simulink model "engine_with_clutch"  (R2026a)
settings: Solver=VariableStepAuto  StopTime=10
libraries: fl_lib x13, nesl_utility x12, sdl_lib x1
settings Model: Creator=doyeop  LastModifiedBy=doyeop
settings SolverCC: ZeroCrossAlgorithm=Adaptive
settings DebuggingCC: IgnoredZcDiagnostic=none

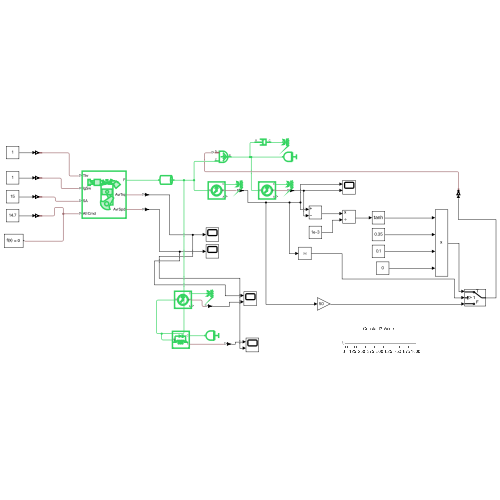
[thumbnail: Simulink's stored preview of the top-level diagram]
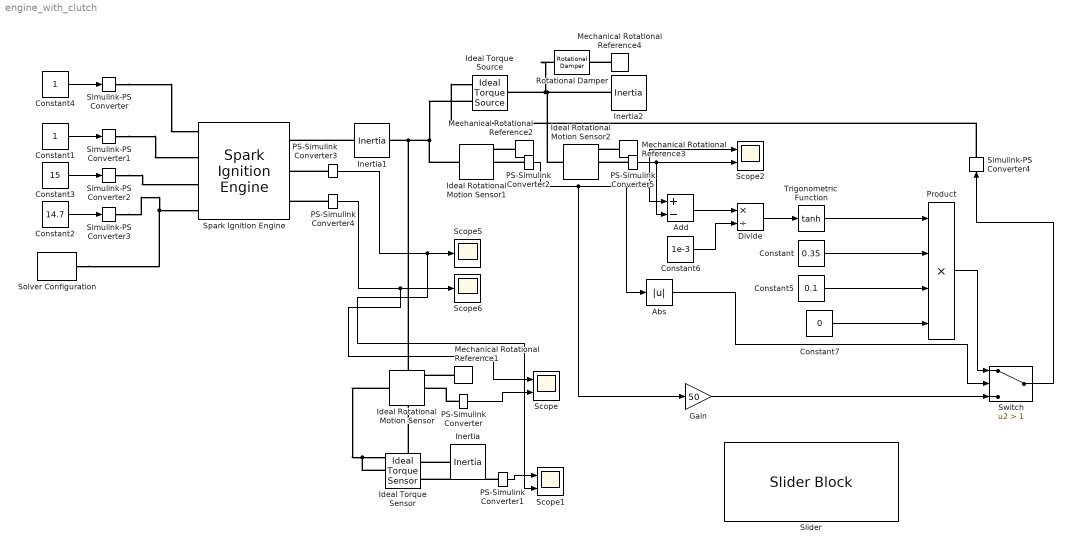
== system engine_with_clutch ==
  Abs : Abs  SaturateOnIntegerOverflow=off
  Add : Sum  Inputs=+-
  Constant : Constant  Value=0.35
  Constant1 : Constant
  Constant2 : Constant  Value=14.7  SampleTime=-1
  Constant3 : Constant  Value=15  SampleTime=-1
  Constant4 : Constant  SampleTime=-1
  Constant5 : Constant  Value=0.1
  Constant6 : Constant  Value=1e-3
  Constant7 : Constant  Value=0
  Divide : Product  Inputs=*/
  Gain : Gain  Gain=50
  Ideal Rotational Motion Sensor : fl_lib/Mechanical/Mechanical Sensors/Ideal Rotational Motion Sensor  reference=foundation.enum.MeasurementReference.difference  acceleration_port=false  velocity_port=true  position_port=true  wrap_angle=false  offset=0 rad
  Ideal Rotational Motion Sensor1 : fl_lib/Mechanical/Mechanical Sensors/Ideal Rotational Motion Sensor  reference=foundation.enum.MeasurementReference.difference  acceleration_port=false  velocity_port=true  position_port=true  wrap_angle=false  offset=0 rad
  Ideal Rotational Motion Sensor2 : fl_lib/Mechanical/Mechanical Sensors/Ideal Rotational Motion Sensor  reference=foundation.enum.MeasurementReference.difference  acceleration_port=false  velocity_port=true  position_port=true  wrap_angle=false  offset=0 rad
  Ideal Torque Sensor : fl_lib/Mechanical/Mechanical Sensors/Ideal Torque Sensor
  Ideal Torque Source : fl_lib/Mechanical/Mechanical Sources/Ideal Torque Source
  Inertia : fl_lib/Mechanical/Rotational Elements/Inertia  inertia=0.1 kg*m^2  num_ports=foundation.enum.numPorts2.one  w_specify=on  w_priority=None  w=0 rpm  w_nominal_specify=off  w_nominal_value=1  w_nominal_unit=rad/s  t_specify=off  t_priority=None  t=0 N*m  t_nominal_specify=off  t_nominal_value=1  t_nominal_unit=N*m
  Inertia1 : fl_lib/Mechanical/Rotational Elements/Inertia  inertia=0.01 kg*m^2  num_ports=foundation.enum.numPorts2.two  w_specify=on  w_priority=High  w=800 rpm  w_nominal_specify=off  w_nominal_value=1  w_nominal_unit=rad/s  t_specify=off  t_priority=None  t=0 N*m  t_nominal_specify=off  t_nominal_value=1  t_nominal_unit=N*m
  Inertia2 : fl_lib/Mechanical/Rotational Elements/Inertia  inertia=0.05 kg*m^2  num_ports=foundation.enum.numPorts2.one  w_specify=on  w_priority=None  w=0 rpm  w_nominal_specify=off  w_nominal_value=1  w_nominal_unit=rad/s  t_specify=off  t_priority=None  t=0 N*m  t_nominal_specify=off  t_nominal_value=1  t_nominal_unit=N*m
  Mechanical Rotational Reference{1..4} (4 alike) : fl_lib/Mechanical/Rotational Elements/Mechanical Rotational Reference
  PS-Simulink Converter{,2,4..5} (4 alike) : nesl_utility/PS-Simulink Converter  PhysicalDomain=network_engine_domain  SubClassName=ps_output  LeftPortType=input  RightPortType=output  PseudoPeriodic=off  Frequencies=[]  VectorFormat=inherit  Unit=rpm  AffineConversion=off
  PS-Simulink Converter1 : nesl_utility/PS-Simulink Converter  PhysicalDomain=network_engine_domain  SubClassName=ps_output  LeftPortType=input  RightPortType=output  PseudoPeriodic=off  Frequencies=[]  VectorFormat=inherit  Unit=N*m  AffineConversion=off
  PS-Simulink Converter3 : nesl_utility/PS-Simulink Converter  PhysicalDomain=network_engine_domain  SubClassName=ps_output  LeftPortType=input  RightPortType=output  PseudoPeriodic=off  Frequencies=[]  VectorFormat=inherit  Unit=N*m  AffineConversion=off
  Product : Product  Inputs=4
  Rotational Damper : fl_lib/Mechanical/Rotational Elements/Rotational Damper  D=0.1 N*m*s/rad  w_specify=off  w_priority=None  w=0 rad/s  w_nominal_specify=off  w_nominal_value=1  w_nominal_unit=rad/s  t_specify=off  t_priority=None  t=0 N*m  t_nominal_specify=off  t_nominal_value=1  t_nominal_unit=N*m
  Scope : Scope  NumInputPorts=2
      settings: ActiveDisplayYMinimum=-2000.3458595498478  ActiveDisplayYMaximum=18003.112735948635
  Scope1 : Scope  NumInputPorts=2
      settings: ActiveDisplayYMinimum=-41.551396950603035  ActiveDisplayYMaximum=102.79160135138113
  Scope2 : Scope  NumInputPorts=2
      settings: ActiveDisplayYMinimum=-1664.2475997401448  ActiveDisplayYMaximum=14978.228397661307  DataLoggingVariableName=ScopeData2
  Scope5 : Scope
      settings: ActiveDisplayYMinimum=-2.7962714720759139  ActiveDisplayYMaximum=25.16644324868323  DataLoggingVariableName=ScopeData5
  Scope6 : Scope
      settings: ActiveDisplayYMinimum=-1506.4519625720234  ActiveDisplayYMaximum=13558.067663148213  DataLoggingVariableName=ScopeData6
  Simulink-PS Converter : nesl_utility/Simulink-PS Converter  PhysicalDomain=network_engine_domain  SubClassName=ps_input  LeftPortType=input  RightPortType=output  PseudoPeriodic=off  Frequencies=[]  NoiseDistribution=none  NoiseParameters=[]  Unit=1  AffineConversion=off  FilteringAndDerivatives=provide  SimscapeFilterOrder=1  InputFilterTimeConstant=0.001  UdotUserProvided=0
  Simulink-PS Converter1 : nesl_utility/Simulink-PS Converter  PhysicalDomain=network_engine_domain  SubClassName=ps_input  LeftPortType=input  RightPortType=output  PseudoPeriodic=off  Frequencies=[]  NoiseDistribution=none  NoiseParameters=[]  Unit=1  AffineConversion=off  FilteringAndDerivatives=provide  SimscapeFilterOrder=1  InputFilterTimeConstant=0.001  UdotUserProvided=0
  Simulink-PS Converter2 : nesl_utility/Simulink-PS Converter  PhysicalDomain=network_engine_domain  SubClassName=ps_input  LeftPortType=input  RightPortType=output  PseudoPeriodic=off  Frequencies=[]  NoiseDistribution=none  NoiseParameters=[]  Unit=deg  AffineConversion=off  FilteringAndDerivatives=provide  SimscapeFilterOrder=1  InputFilterTimeConstant=0.001  UdotUserProvided=0
  Simulink-PS Converter3 : nesl_utility/Simulink-PS Converter  PhysicalDomain=network_engine_domain  SubClassName=ps_input  LeftPortType=input  RightPortType=output  PseudoPeriodic=off  Frequencies=[]  NoiseDistribution=none  NoiseParameters=[]  Unit=1  AffineConversion=off  FilteringAndDerivatives=provide  SimscapeFilterOrder=1  InputFilterTimeConstant=0.001  UdotUserProvided=0
  Simulink-PS Converter4 : nesl_utility/Simulink-PS Converter  PhysicalDomain=network_engine_domain  SubClassName=ps_input  LeftPortType=input  RightPortType=output  PseudoPeriodic=off  Frequencies=[]  NoiseDistribution=none  NoiseParameters=[]  Unit=1  AffineConversion=off  FilteringAndDerivatives=filter  SimscapeFilterOrder=1  InputFilterTimeConstant=1e-3  UdotUserProvided=0
  Slider : SliderBlock  ScaleMax=1000
  Solver Configuration : nesl_utility/Solver Configuration  PhysicalDomain=network_engine_domain  SubClassName=solver  LeftPortType=input  RightPortType=generic  Tones=[]  Harmonics=[]  SimulateNoise=off  Profile=off  UseLocalSampling=off  EnableSwitchedLinearOptims=on  FrequencyDomain=off  UseCCode=off  RelTol=0.001  AbsTol=0.001  MinStep=1e-09  ToWorkspace=off  RevertToSquareIcSolve=off  NumHomotopyIterations=100  PhasorMode=off  PhasorModeNumHarmonics=1  ConsistencySolver=NEWTON_XTOL_AFTER_FTOL  CanonicalOrdering=CANONICAL  OptimizeIntermediates=OPTIMIZED  IndexReductionMethod=DerivativeReplacement  DoDC=off  ResidualTolerance=1e-09  ConsistencyTolSource=GLOBAL  ConsistencyAbsTol=0.001  ConsistencyRelTol=0.001  ConsistencyTolFactor=0.001  UseLocalSolver=off  LocalSolverChoice=NE_BACKWARD_EULER_ADVANCER  ResolveIndetEquations=on  FunctionEvalNumThread=1  LocalSolverSampleTime=0.001  DoFixedCost=off  MaxNonlinIter=3  MaxModeIter=2  ComputeImpulses=off  ImpulseIterations=2  LinearAlgebra=auto  LinearAlgebraNumThread=0  EquationFormulation=NE_TIME_EF  DelaysMemoryBudget=1024  AutomaticFiltering=on  FilteringTimeConstant=0.001  PartitionStorageMethod=AS_NEEDED  PartitionMemoryBudget=1024  PartitionMethod=ROBUST  MultibodyUseLocalSolver=off  MultibodyLocalSolverChoice=ODE1  MultibodyLocalSolverSampleTime=0.001
  Spark Ignition Engine : sdl_lib/Engines & Motors/Spark Ignition Engine  numCyls=sdl.enum.engineNumCylinders.Four  twoCylSADiff=270 deg  L4FiringOrder=sdl.enum.engineFiringOrderFourCylinders.L4_1342  bore=67 mm  stroke=42.5 mm  conrod=90 mm  CR=12.2  P_amb=101.325 kPa  T_amb=298.15 K  rho_air=1.225 mg/cm^3  R_air=288.1965 J/(K*kg)  UseAirIntake=true  c_thr=0.1 s  thr_rest=3 deg  D_plate=5 cm  S_leak=1 cm^2  V_im=500 cm^3  Cd_in=0.9  IVO_0=-10 deg  IVC_0=100 deg  EVO_0=30 deg  EVC_0=5 deg  UseInVVT=false  UseExVVT=false  q_LHV=44.3 MJ/kg  InputAFR=true  AFR_const=14.6  InputInjPw=false  Sinj=6.5 mg/ms  SparkInputType=sdl.enum.engineSparkInputType.Angle  SA_const=20 deg  comb_bd=50 deg  dt_Pcyl_slow_decay=60 s  dt_Tcyl_slow_decay=600 s  dt_exh_decay=5 ms  InputBackPressure=false  dP_exh=50 kPa  dw_exh=6000 rpm  UseExhaustThermal=true  S_exh=1 m^2  M_exh=5 kg  C_exh=100 J/(K*kg)  k_gas=10 s  h_convection=100 W/(K*m^2)  k_radiation=0.3  SB=5.7e-8 W/(K^4*m^2)  Pim_0=101.325 kPa  ca0=0 deg  w0=800 rpm  EngSpdSimLimit=16000 rpm  OutputTorqueAvr=true  OutputSpeedAvr=true  OutputCrkpos=false  OutputPim=false  OutputAirMassFlow=false  OutputFuelMassFlow=false  OutputAFR=false  OutputVcyl=false  OutputPcyl=false  OutputTcyl=false  OutputTexh=false
  Switch : Switch  Criteria=u2 > Threshold  Threshold=1  SaturateOnIntegerOverflow=off  InputSameDT=off
  Trigonometric Function : Trigonometry  Operator=tanh
  wires:
  Constant4/1 -> Simulink-PS Converter/1
  Constant1/1 -> Simulink-PS Converter1/1
  Constant3/1 -> Simulink-PS Converter2/1
  Constant2/1 -> Simulink-PS Converter3/1
  PS-Simulink Converter3/1 -> Scope1/2, Scope5/1
  PS-Simulink Converter4/1 -> Scope/1, Scope6/1
  PS-Simulink Converter/1 -> Scope/2
  PS-Simulink Converter1/1 -> Scope1/1
  PS-Simulink Converter2/1 -> Gain/1, Abs/1, Scope2/1, Add/1
  PS-Simulink Converter5/1 -> Add/2, Scope2/2
  Add/1 -> Divide/1
  Trigonometric Function/1 -> Product/1
  Constant/1 -> Product/2
  Constant5/1 -> Product/3
  Gain/1 -> Switch/3
  Constant6/1 -> Divide/2
  Divide/1 -> Trigonometric Function/1
  Product/1 -> Switch/1
  Abs/1 -> Switch/2
  Switch/1 -> Simulink-PS Converter4/1
  Constant7/1 -> Product/4
  connections:
  Simulink-PS Converter/RConn1 -- Spark Ignition Engine/LConn1
  Simulink-PS Converter1/RConn1 -- Spark Ignition Engine/LConn2
  Simulink-PS Converter2/RConn1 -- Spark Ignition Engine/LConn3
  Simulink-PS Converter3/RConn1 -- Solver Configuration/RConn1 -- Spark Ignition Engine/LConn4
  Inertia1/RConn1 -- Spark Ignition Engine/RConn1
  PS-Simulink Converter/LConn1 -- Ideal Rotational Motion Sensor/RConn2
  PS-Simulink Converter1/LConn1 -- Ideal Torque Sensor/RConn2
  Mechanical Rotational Reference1/LConn1 -- Ideal Rotational Motion Sensor/RConn1
  PS-Simulink Converter3/LConn1 -- Spark Ignition Engine/RConn2
  PS-Simulink Converter4/LConn1 -- Spark Ignition Engine/RConn3
  Inertia/LConn1 -- Ideal Torque Sensor/RConn1
  Ideal Torque Source/RConn2 -- Ideal Rotational Motion Sensor1/LConn1 -- Ideal Torque Sensor/LConn1 -- Ideal Rotational Motion Sensor/LConn1 -- Inertia1/LConn1
  Inertia2/LConn1 -- Ideal Rotational Motion Sensor2/LConn1 -- Rotational Damper/LConn1 -- Ideal Torque Source/LConn1
  PS-Simulink Converter2/LConn1 -- Ideal Rotational Motion Sensor1/RConn2
  PS-Simulink Converter5/LConn1 -- Ideal Rotational Motion Sensor2/RConn2
  Simulink-PS Converter4/RConn1 -- Ideal Torque Source/RConn1
  Mechanical Rotational Reference2/LConn1 -- Ideal Rotational Motion Sensor1/RConn1
  Mechanical Rotational Reference3/LConn1 -- Ideal Rotational Motion Sensor2/RConn1
  Mechanical Rotational Reference4/LConn1 -- Rotational Damper/RConn1
